simulink model "drone_estimator_angle_dynamics"  (R2024a)
settings: Solver=FixedStepAuto  StartTime=0.0  StopTime=30  FixedStep=0.001  RelTol=1e-3
InitFcn:
  | os = 0.15;
  | zeta = -log(os)/sqrt(pi^2+(log(os))^2);
  | ts = 0.2;
  | wn = 4/zeta/ts;
  | kx = wn^2 - 1;
  | kf = 2 * zeta * wn;
  | Kx = eye(2) * kx;
  | Kf = eye(2) * kf;
  | 
  | 
  | os_des = 0.1;
  | zeta_des = -log(os_des)/sqrt(pi^2+(log(os_des))^2);
  | ts_des = 1;
  | wn_des = 4/zeta_des/ts_des;
  | b_des = wn_des^2;
  | a_des = 2 * zeta_des * wn_des;
undefined symbols (not defined in the file or in its folder): e0_0, e1_0, e2_0, e3_0, q0, QP, vec
libraries: sharedtransform x12, dspsigops x12, sharedutil x6, simulink x3
(part 1 of 2)
settings Model: Creator=bemran  LastModifiedBy=bemran

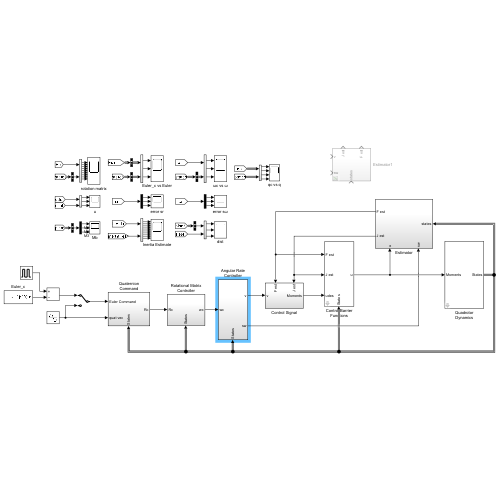
[thumbnail: Simulink's stored preview of the top-level diagram]
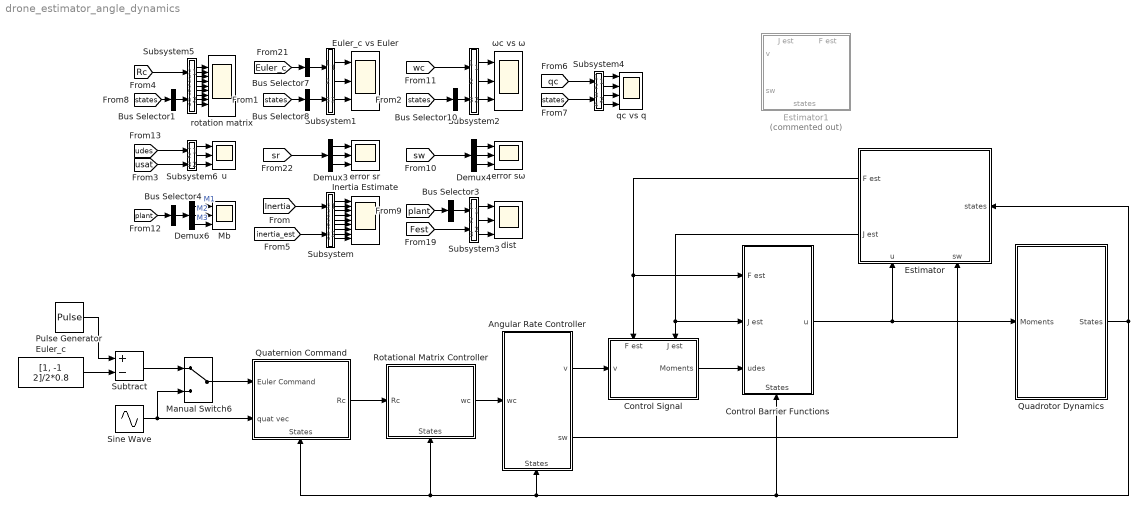
== system drone_estimator_angle_dynamics ==
  Angular Rate Controller : Subsystem
      settings: PortSchema="{\"entries\":[{\"content\":{\"sides\":[{\"content\":{\"connectorIds\":[\"In1\"]},\"type\":\"ConnectorPlacement.EquallySpacedRectSide\",\"uuid\":\"bc172b6d-1998-4b63-a77e-55c15233d681\"},{\"content\":{\"connectorIds\":[\"Out1\",\"Out2\"],\"side\":\"RIGHT\"},\"type\":\"ConnectorPlacement.EquallySpacedRectSide\",\"uuid\":\"e273a2d7-8de6-43d9-a3cd-224a066eb420\"},{\"content\":{\"side\":\"TOP\"},\"type\":\"ConnectorPlacement.EquallySpacedRectSide\",\"uuid\":\"072f3d67-5acb-4515-8061-1025c18e9c92\"},{\"content\":{\"connectorIds\":[\"In2\"],\"side\":\"BOTTOM\"},\"type\":\"ConnectorPlacement.EquallySpacedRectSide\",\"uuid\":\"23d2cd87-0863-4bc6-9ec0-2d909e89db59\"}]},\"type\":\"ConnectorPlacement.EquallySpacedConnector\",\"uuid\":\"0291006e-df7f-48c2-854b-3fa02a3c9ebe\"}],\"packageUris\":[\"http://schema.mathworks.com/mf0/Connector/R2020b\"],\"version\":\"1.0\"}"
  Bus Selector1 : BusSelector  OutputSignals=DCM_be  OutputAsBus=on
  Bus Selector10 : BusSelector  OutputSignals=w.p,w.q,w.r  OutputAsBus=on
  Bus Selector3 : BusSelector  OutputSignals=dist  OutputAsBus=on
  Bus Selector4 : BusSelector  OutputSignals=u  OutputAsBus=on
  Bus Selector7 : BusSelector  OutputSignals=ϕc,θc,Ψc  OutputAsBus=on
  Bus Selector8 : BusSelector  OutputSignals=Euler.ϕ,Euler.θ,Euler.Ψ  OutputAsBus=on
  Control Barrier Functions : Subsystem  mask{MaxU=30, MinU=-30, MaxW=20, MinW=-20}
      mask prompts: MaxU "Maximum Momentum"; MinU "Minimum Momentum"; MaxW "Maximum Omega"; MinW "Minimum Omega"
      settings: PortSchema="{\"entries\":[{\"content\":{\"sides\":[{\"content\":{\"connectorIds\":[\"In1\",\"In2\",\"In3\"]},\"type\":\"ConnectorPlacement.EquallySpacedRectSide\",\"uuid\":\"dcc8a69e-9139-493e-8673-5f35c41b34de\"},{\"content\":{\"connectorIds\":[\"Out1\"],\"side\":\"RIGHT\"},\"type\":\"ConnectorPlacement.EquallySpacedRectSide\",\"uuid\":\"2dca4313-3691-4a08-9138-e65173157107\"},{\"content\":{\"side\":\"TOP\"},\"type\":\"ConnectorPlacement.EquallySpacedRectSide\",\"uuid\":\"349ab802-a657-4b93-842b-98d2d831e594\"},{\"content\":{\"connectorIds\":[\"In4\"],\"side\":\"BOTTOM\"},\"type\":\"ConnectorPlacement.EquallySpacedRectSide\",\"uuid\":\"8ea90ba3-5825-4aab-a654-9f2643502d53\"}]},\"type\":\"ConnectorPlacement.EquallySpacedConnector\",\"uuid\":\"4208f7a9-c52c-44b5-9388-6b2af73cf8e5\"}],\"packageUris\":[\"http://schema.mathworks.com/mf0/Connector/R2020b\"],\"version\":\"1.0\"}"
      mask TypeOptions MaxU: MaxU/Value
      mask TypeOptions MinU: MinU/Value
      mask TypeOptions MaxW: MaxW/Value
      mask TypeOptions MinW: MinW/Value
  Control Signal : Subsystem
      settings: PortSchema="{\"entries\":[{\"content\":{\"sides\":[{\"content\":{\"connectorIds\":[\"In1\"]},\"type\":\"ConnectorPlacement.EquallySpacedRectSide\",\"uuid\":\"8e76b4e0-9a75-4e0d-89ba-89445e2fc413\"},{\"content\":{\"connectorIds\":[\"Out1\"],\"side\":\"RIGHT\"},\"type\":\"ConnectorPlacement.EquallySpacedRectSide\",\"uuid\":\"8c2e0e8a-5733-437d-85b2-5dcae92259bc\"},{\"content\":{\"connectorIds\":[\"In2\",\"In3\"],\"side\":\"TOP\"},\"type\":\"ConnectorPlacement.EquallySpacedRectSide\",\"uuid\":\"0f355bac-c390-4b16-a489-c47462c0e821\"},{\"content\":{\"side\":\"BOTTOM\"},\"type\":\"ConnectorPlacement.EquallySpacedRectSide\",\"uuid\":\"c09fe95f-7587-46e4-92c1-9bab0ec13c57\"}]},\"type\":\"ConnectorPlacement.EquallySpacedConnector\",\"uuid\":\"5b127af5-2db1-4950-aad7-ca3070de8172\"}],\"packageUris\":[\"http://schema.mathworks.com/mf0/Connector/R2020b\"],\"version\":\"1.0\"}"
  Demux3 : Demux  Outputs=3
  Demux4 : Demux  Outputs=3
  Demux6 : Demux  Outputs=3
  Estimator : Subsystem
      settings: PortSchema="{\"entries\":[{\"content\":{\"sides\":[{\"content\":{},\"type\":\"ConnectorPlacement.EquallySpacedRectSide\",\"uuid\":\"dd8d0a7b-0398-466a-94a7-19864dbb7504\"},{\"content\":{\"connectorIds\":[\"In2\",\"In3\"],\"side\":\"RIGHT\"},\"type\":\"ConnectorPlacement.EquallySpacedRectSide\",\"uuid\":\"1f79f4fb-283e-4db7-838d-a1872a06439d\"},{\"content\":{\"connectorIds\":[\"In1\"],\"side\":\"TOP\"},\"type\":\"ConnectorPlacement.EquallySpacedRectSide\",\"uuid\":\"5e0e8233-da53-4403-9876-3f6f01163ba4\"},{\"content\":{\"connectorIds\":[\"Out1\",\"Out2\"],\"side\":\"BOTTOM\"},\"type\":\"ConnectorPlacement.EquallySpacedRectSide\",\"uuid\":\"ef1fb064-42c9-4e33-ac14-a7a48f45da2d\"}]},\"type\":\"ConnectorPlacement.EquallySpacedConnector\",\"uuid\":\"c21bdc57-4e96-4c86-bff3-633ae446dfd3\"}],\"packageUris\":[\"http://schema.mathworks.com/mf0/Connector/R2020b\"],\"version\":\"1.0\"}"
  Estimator1 : Subsystem  Commented=on
      settings: PortSchema="{\"entries\":[{\"content\":{\"sides\":[{\"content\":{\"connectorIds\":[\"In1\",\"In2\"]},\"type\":\"ConnectorPlacement.EquallySpacedRectSide\",\"uuid\":\"dd8d0a7b-0398-466a-94a7-19864dbb7504\"},{\"content\":{\"side\":\"RIGHT\"},\"type\":\"ConnectorPlacement.EquallySpacedRectSide\",\"uuid\":\"1f79f4fb-283e-4db7-838d-a1872a06439d\"},{\"content\":{\"connectorIds\":[\"Out1\",\"Out2\"],\"side\":\"TOP\"},\"type\":\"ConnectorPlacement.EquallySpacedRectSide\",\"uuid\":\"5e0e8233-da53-4403-9876-3f6f01163ba4\"},{\"content\":{\"connectorIds\":[\"In3\"],\"side\":\"BOTTOM\"},\"type\":\"ConnectorPlacement.EquallySpacedRectSide\",\"uuid\":\"ef1fb064-42c9-4e33-ac14-a7a48f45da2d\"}]},\"type\":\"ConnectorPlacement.EquallySpacedConnector\",\"uuid\":\"c21bdc57-4e96-4c86-bff3-633ae446dfd3\"}],\"packageUris\":[\"http://schema.mathworks.com/mf0/Connector/R2020b\"],\"version\":\"1.0\"}"
  Euler_c : Constant  Value=[1, -1 2]/2*0.8
  Euler_c vs Euler : Scope  NumInputPorts=3
  Inertia Estimate : Scope  NumInputPorts=9
  Manual Switch6 : ManualSwitch
  Mb : Scope  NumInputPorts=3
  Pulse Generator : DiscretePulseGenerator  PulseType=Time based  Amplitude=[-1, -1, 4]*0.8  Period=[25, 37, 45]  PulseWidth=[60, 40, 50]  PhaseDelay=[0, 13, 8]
  Quadrotor Dynamics : Subsystem  mask{InertiaM=[1.7, 0.2, 0.3; 0.2, 2.4, 0.7; 0.3, 0.7, 3.2] + [QP.InertiaMatrix * 0 + diag([1.5,1.2,2]) + ones(3)*0.2]*0, EulerInitialValues=[1, 0.8, 1]*-pi/2, OmegaInitialValues=[-1;1; 1]*-1}
      mask prompts: InertiaM "Inertia Matrix"; EulerInitialValues "Euler Initial Values"; OmegaInitialValues "Omega Initial Values"
      mask TypeOptions InertiaM: Dynamics/Angular Velocity Dyanmics/InertiaMatrix
      mask TypeOptions EulerInitialValues: Dynamics/Quaternion Dynamics/EulerInitialValues
      mask TypeOptions OmegaInitialValues: Dynamics/Angular Velocity Dyanmics/OmegaInitialValues
      mask DialogControl Container4 Prompt: Parameters
      mask DialogControl Container5 Prompt: Initial Conditions
  Quaternion Command : Subsystem
      settings: PortSchema="{\"entries\":[{\"content\":{\"sides\":[{\"content\":{\"connectorIds\":[\"In1\",\"In2\"]},\"type\":\"ConnectorPlacement.EquallySpacedRectSide\",\"uuid\":\"ab38e5a5-80b4-4ab8-a53a-65892619af31\"},{\"content\":{\"connectorIds\":[\"Out1\"],\"side\":\"RIGHT\"},\"type\":\"ConnectorPlacement.EquallySpacedRectSide\",\"uuid\":\"8715b2e2-d98c-47a7-9943-c760a43dac77\"},{\"content\":{\"side\":\"TOP\"},\"type\":\"ConnectorPlacement.EquallySpacedRectSide\",\"uuid\":\"40574ceb-ae4a-44b3-ac35-a21b012f7856\"},{\"content\":{\"connectorIds\":[\"In3\"],\"side\":\"BOTTOM\"},\"type\":\"ConnectorPlacement.EquallySpacedRectSide\",\"uuid\":\"26ed6dc8-3652-4856-a0a2-f0a897d5f128\"}]},\"type\":\"ConnectorPlacement.EquallySpacedConnector\",\"uuid\":\"d4d113a2-0092-45e8-ae58-dde56ef36bed\"}],\"packageUris\":[\"http://schema.mathworks.com/mf0/Connector/R2020b\"],\"version\":\"1.0\"}"
  Rotational Matrix Controller : Subsystem
      settings: PortSchema="{\"entries\":[{\"content\":{\"sides\":[{\"content\":{\"connectorIds\":[\"In1\"]},\"type\":\"ConnectorPlacement.EquallySpacedRectSide\",\"uuid\":\"3d78e969-c8a0-4bae-8d29-4309eff7c33e\"},{\"content\":{\"connectorIds\":[\"Out1\"],\"side\":\"RIGHT\"},\"type\":\"ConnectorPlacement.EquallySpacedRectSide\",\"uuid\":\"5a76abcf-08d0-4f78-ba00-cefe271d19f3\"},{\"content\":{\"side\":\"TOP\"},\"type\":\"ConnectorPlacement.EquallySpacedRectSide\",\"uuid\":\"9a4251fd-9b0c-42f6-8a3e-81b1fbae2b4d\"},{\"content\":{\"connectorIds\":[\"In2\"],\"side\":\"BOTTOM\"},\"type\":\"ConnectorPlacement.EquallySpacedRectSide\",\"uuid\":\"0ec39cec-73e3-40ef-a15f-c71162c87a73\"}]},\"type\":\"ConnectorPlacement.EquallySpacedConnector\",\"uuid\":\"a6a66122-20c0-4355-ae71-2ed9e39c6f14\"}],\"packageUris\":[\"http://schema.mathworks.com/mf0/Connector/R2020b\"],\"version\":\"1.0\"}"
  Sine Wave : Sin  Amplitude=[1*pi;1*pi; 1*pi]/2  Frequency=[0.1, 0.05, 0.02]  Phase=[pi/6, pi/2, -pi/6]  SampleTime=0
  Subsystem : Subsystem
  Subsystem1 : Subsystem
  Subsystem2 : Subsystem
  Subsystem3 : Subsystem
  Subsystem4 : Subsystem
  Subsystem5 : Subsystem
  Subsystem6 : Subsystem
  Subtract : Sum  Inputs=+-
  dist : Scope  NumInputPorts=3
  error sr : Scope  NumInputPorts=3
  error sω : Scope  NumInputPorts=3
  qc vs q : Scope  NumInputPorts=4
  rotation matrix : Scope  NumInputPorts=9
  u : Scope  NumInputPorts=3
  ωc vs ω : Scope  NumInputPorts=3
  wires:
  Quaternion Command/1(Rc) -> Rotational Matrix Controller/1(Rc)
  Control Barrier Functions/1(u) -> Estimator/3(u), Quadrotor Dynamics/1(Moments)
  [sr] -> Demux3/1
  [states] -> Bus Selector10/1
  Subsystem2/1(Out1) -> ωc vs ω/1
  [wc] -> Subsystem2/1(wc)
  Demux6/3 -> Mb/3  "M3"
  Demux6/1 -> Mb/1  "M1"
  Demux6/2 -> Mb/2  "M2"
  Demux4/1 -> error sω/1
  Subsystem2/3(Out3) -> ωc vs ω/3
  [sw] -> Demux4/1
  Demux3/1 -> error sr/1
  Demux4/2 -> error sω/2
  Subsystem2/2(Out2) -> ωc vs ω/2
  Demux3/2 -> error sr/2
  Bus Selector4/1 -> Demux6/1
  Demux3/3 -> error sr/3
  Demux4/3 -> error sω/3
  [Fest] -> Subsystem3/2(fest)
  Subsystem3/1(Out1) -> dist/1
  Subsystem3/3(Out3) -> dist/3
  Subsystem3/2(Out2) -> dist/2
  [plant] -> Bus Selector3/1
  Control Signal/1(Moments) -> Control Barrier Functions/3(udes)
  Subsystem/1(Out1) -> Inertia Estimate/1
  Subsystem/2(Out2) -> Inertia Estimate/2
  Subsystem/3(Out3) -> Inertia Estimate/3
  Subsystem/4(Out4) -> Inertia Estimate/4
  Subsystem/5(Out5) -> Inertia Estimate/5
  Subsystem/6(Out6) -> Inertia Estimate/6
  Subsystem/7(Out7) -> Inertia Estimate/7
  Subsystem/8(Out8) -> Inertia Estimate/8
  Subsystem/9(Out9) -> Inertia Estimate/9
  [inertia_est] -> Subsystem/2(In6)
  [Euler_c] -> Bus Selector7/1
  [states] -> Bus Selector8/1
  Subsystem1/1(Out1) -> Euler_c vs Euler/1
  Subsystem1/2(Out2) -> Euler_c vs Euler/2
  Subsystem1/3(Out3) -> Euler_c vs Euler/3
  Bus Selector7/1 -> Subsystem1/1(Euler_c)
  Bus Selector8/1 -> Subsystem1/2(Euler)
  Bus Selector10/1 -> Subsystem2/2(w)
  Euler_c/1 -> Subtract/2
  Pulse Generator/1 -> Subtract/1
  Manual Switch6/1 -> Quaternion Command/1(Euler Command)
  Subtract/1 -> Manual Switch6/1
  Subsystem4/2(Out2) -> qc vs q/2
  Subsystem4/3(Out3) -> qc vs q/3
  [qc] -> Subsystem4/1(In1)
  Subsystem4/1(Out1) -> qc vs q/1
  [states] -> Subsystem4/2(In3)
  Subsystem4/4(Out4) -> qc vs q/4
  [states] -> Bus Selector1/1
  [Rc] -> Subsystem5/1(In4)
  Subsystem5/9(Out9) -> rotation matrix/9
  Subsystem5/8(Out8) -> rotation matrix/8
  Subsystem5/7(Out7) -> rotation matrix/7
  Subsystem5/6(Out6) -> rotation matrix/6
  Subsystem5/5(Out5) -> rotation matrix/5
  Subsystem5/4(Out4) -> rotation matrix/4
  Subsystem5/3(Out3) -> rotation matrix/3
  Subsystem5/2(Out2) -> rotation matrix/2
  Subsystem5/1(Out1) -> rotation matrix/1
  Bus Selector1/1 -> Subsystem5/2(In6)
  [Inertia] -> Subsystem/1(In4)
  Bus Selector3/1 -> Subsystem3/1(dist)
  [plant] -> Bus Selector4/1
  Sine Wave/1 -> Manual Switch6/2, Quaternion Command/2(quat vec)
  Estimator/2(J est) -> Control Signal/3(J est), Control Barrier Functions/2(J est)
  Estimator/1(F est) -> Control Signal/2(F est), Control Barrier Functions/1(F est)
  Rotational Matrix Controller/1(wc) -> Angular Rate Controller/1(wc)
  Quadrotor Dynamics/1(States) -> Estimator/1(states), Quaternion Command/3(States), Rotational Matrix Controller/2(States), Angular Rate Controller/2(States), Control Barrier Functions/4(States)
  Angular Rate Controller/1(v) -> Control Signal/1(v)
  Angular Rate Controller/2(sw) -> Estimator/2(sw)
  [usat] -> Subsystem6/2(u sat)
  Subsystem6/1(Out1) -> u/1
  Subsystem6/2(Out2) -> u/2
  Subsystem6/3(Out3) -> u/3
  [udes] -> Subsystem6/1(u)

== system drone_estimator_angle_dynamics/Angular Rate Controller ==
  wc : Inport
  In Bus Element : Inport  Port=2  PortName=States  Element=w
  Add : Sum
  Dynamic Surface Angular Rate Controller : Subsystem  mask{OmegaTimeConstant=20, PControllerGain=9, IControllerGain=4, DesiredAngularRateInitCond=zeros(3,1)}
      mask prompts: OmegaTimeConstant "Omega Time Constant"; PControllerGain "Propotional Controller Gain"; IControllerGain "Integral Controller Gain"; DesiredAngularRateInitCond "Desired Angular Rate Initial Condition"
      mask TypeOptions OmegaTimeConstant:
      | Angular Rate
      | Desired Dynamics/tau/Gain
      mask TypeOptions PControllerGain: P gain/Gain
      mask TypeOptions IControllerGain: I gain/Gain
      mask TypeOptions DesiredAngularRateInitCond:
      | Angular Rate
      | Desired Dynamics/Desired Angular
      | Rate Integaration/InitialCondition
  Manual Switch : ManualSwitch  CurrentSetting=0
  Pulse Generator : DiscretePulseGenerator  PulseType=Time based  Amplitude=[3, -3, 3]*0.8  Period=[20, 20, 20]  PulseWidth=50  PhaseDelay=[0 7 13]
  Sine Wave : Sin  Amplitude=[1*pi;1*pi; 1*pi]  Frequency=[0.1, 0.05, 0.02]*10  Phase=[pi/6, pi/2, -pi/6]  SampleTime=0
  v : Outport
  sw : Outport  Port=2
  wires:
  Sine Wave/1 -> Add/2
  Manual Switch/1 -> Dynamic Surface Angular Rate Controller/1(wc)
  Dynamic Surface Angular Rate Controller/2(sw) -> sw/1
  Pulse Generator/1 -> Add/1
  Dynamic Surface Angular Rate Controller/1(v) -> v/1
  Add/1 -> Manual Switch/1
  wc/1 -> Manual Switch/2
  In Bus Element/1 -> Dynamic Surface Angular Rate Controller/2(w)

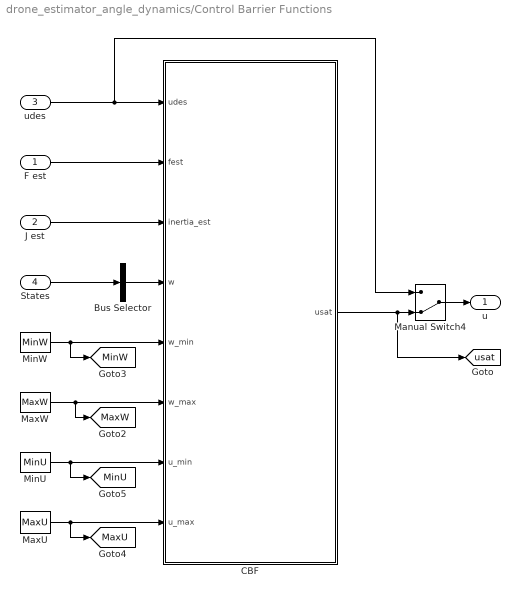
== system drone_estimator_angle_dynamics/Control Barrier Functions ==
  F est : Inport
  J est : Inport  Port=2
  udes : Inport  Port=3
  States : Inport  Port=4
  Bus Selector : BusSelector  OutputSignals=w.p,w.q,w.r  OutputAsBus=on
  CBF : MATLAB Function  TreatAsAtomicUnit=on
  Manual Switch4 : ManualSwitch  CurrentSetting=0
  MaxU : Constant  Value=MaxU
  MaxW : Constant  Value=MaxW
  MinU : Constant  Value=MinU
  MinW : Constant  Value=MinW
  u : Outport
  tag scope: MaxU=global, MaxW=global, MinU=global, MinW=global, usat=global
  wires:
  J est/1 -> CBF/3(inertia_est)
  MaxW/1 -> [MaxW], CBF/6(w_max)
  MinW/1 -> [MinW], CBF/5(w_min)
  F est/1 -> CBF/2(fest)
  MinU/1 -> [MinU], CBF/7(u_min)
  MaxU/1 -> [MaxU], CBF/8(u_max)
  Bus Selector/1 -> CBF/4(w)
  States/1 -> Bus Selector/1
  CBF/1(usat) -> [usat], Manual Switch4/2
  udes/1 -> Manual Switch4/1, CBF/1(udes)
  Manual Switch4/1 -> u/1

== system drone_estimator_angle_dynamics/Control Signal ==
  v : Inport
  F est : Inport  Port=2
  J est : Inport  Port=3
  Product : Product  Inputs=**  Multiplication=Matrix(*)
  Sum1 : Sum  Inputs=|+-
  Moments : Outport
  tag scope: udes=global
  wires:
  Sum1/1 -> [udes], Moments/1
  F est/1 -> Sum1/2
  Product/1 -> Sum1/1
  v/1 -> Product/2
  J est/1 -> Product/1

== system drone_estimator_angle_dynamics/Estimator ==
  states : Inport
  sw : Inport  Port=2
  u : Inport  Port=3
  Add : Sum
  Constant : Constant  Value=zeros(3,1)
  Gain : Gain  Gain=0.3
  Inertia Estimation : Subsystem  mask{gamma=QP.InertiaMatrixGamma*5, MaxEstiamtedTheta=QP.InertiaMatrixMax*0 + 3*eye(3) + ones(3), MinEstiamtedTheta=QP.InertiaMatrixMin*0 + eye(3)*0.01, eps=0.01, InertiaInitialCondition=eye(3) + ones(3)*0.1}
      mask prompts: MaxEstiamtedTheta "Maximum Estiamted Theta"; MinEstiamtedTheta "Minimum Estiamted Theta"; eps "Epsilon Estiamted Theta"; InertiaInitialCondition "Inertia Initial Condition"
      mask TypeOptions gamma: gama/Gain
      mask TypeOptions MaxEstiamtedTheta: θ Max/Value
      mask TypeOptions MinEstiamtedTheta: θ Min/Value
      mask TypeOptions eps: eps/Value
      mask TypeOptions InertiaInitialCondition: θ estimate/InitialCondition
      mask DialogControl Container Prompt: Estimation Paraemter
  Manual Switch : ManualSwitch
  Manual Switch1 : ManualSwitch  CurrentSetting=0
  Model Predictor : Subsystem
      settings: PortSchema="{\"entries\":[{\"content\":{\"sides\":[{\"content\":{\"connectorIds\":[\"Out1\",\"Out2\"]},\"type\":\"ConnectorPlacement.EquallySpacedRectSide\",\"uuid\":\"6e6569c2-bc7f-4167-ae98-e66125c9e1e3\"},{\"content\":{\"connectorIds\":[\"In1\",\"In2\",\"In3\"],\"side\":\"RIGHT\"},\"type\":\"ConnectorPlacement.EquallySpacedRectSide\",\"uuid\":\"af0deaad-808c-4137-9b9d-c847525b3dac\"},{\"content\":{\"side\":\"TOP\"},\"type\":\"ConnectorPlacement.EquallySpacedRectSide\",\"uuid\":\"ed017cdd-fa89-4299-a174-caff2025e69e\"}]},\"type\":\"ConnectorPlacement.EquallySpacedConnector\",\"uuid\":\"feb2a9a1-0b16-4155-b32e-177a30695464\"}],\"packageUris\":[\"http://schema.mathworks.com/mf0/Connector/R2020b\"],\"version\":\"1.0\"}"
  Model Predictor1 : Subsystem  Commented=on
      settings: PortSchema="{\"entries\":[{\"content\":{\"sides\":[{\"content\":{\"connectorIds\":[\"Out1\",\"Out2\"]},\"type\":\"ConnectorPlacement.EquallySpacedRectSide\",\"uuid\":\"6e6569c2-bc7f-4167-ae98-e66125c9e1e3\"},{\"content\":{\"connectorIds\":[\"In1\",\"In2\",\"In3\",\"In4\"],\"side\":\"RIGHT\"},\"type\":\"ConnectorPlacement.EquallySpacedRectSide\",\"uuid\":\"af0deaad-808c-4137-9b9d-c847525b3dac\"},{\"content\":{\"side\":\"TOP\"},\"type\":\"ConnectorPlacement.EquallySpacedRectSide\",\"uuid\":\"ed017cdd-fa89-4299-a174-caff2025e69e\"}]},\"type\":\"ConnectorPlacement.EquallySpacedConnector\",\"uuid\":\"feb2a9a1-0b16-4155-b32e-177a30695464\"}],\"packageUris\":[\"http://schema.mathworks.com/mf0/Connector/R2020b\"],\"version\":\"1.0\"}"
  F est : Outport
  J est : Outport  Port=2
  tag scope: inertia_est=global
  wires:
  Model Predictor/1(er) -> Add/1
  Inertia Estimation/1("  θ est") -> Manual Switch/1
  [Inertia] -> Manual Switch/2
  Model Predictor/2(F est) -> F est/1
  Manual Switch/1 -> Model Predictor/3(J est), [inertia_est], J est/1
  states/1 -> Model Predictor/1(x)
  u/1 -> Model Predictor/2(u), Inertia Estimation/1(u)
  sw/1 -> Gain/1
  Gain/1 -> Manual Switch1/2
  Constant/1 -> Manual Switch1/1
  Manual Switch1/1 -> Add/2
  Add/1 -> Inertia Estimation/2(e)

== system drone_estimator_angle_dynamics/Estimator1 ==
  v : Inport
  sw : Inport  Port=2
  states : Inport  Port=3
  Add : Sum
  Constant : Constant  Value=zeros(3,1)
  Gain : Gain  Gain=0.3
  Inertia Estimation : Subsystem  mask{gamma=QP.InertiaMatrixGamma*1, MaxEstiamtedTheta=QP.InertiaMatrixMax*0 + 3*eye(3) + ones(3)*0.5, MinEstiamtedTheta=QP.InertiaMatrixMin*0 + eye(3)*0.01, eps=0.01, InertiaInitialCondition=ones(3)*0.3 + eye(3)}
      mask prompts: MaxEstiamtedTheta "Maximum Estiamted Theta"; MinEstiamtedTheta "Minimum Estiamted Theta"; eps "Epsilon Estiamted Theta"; InertiaInitialCondition "Inertia Initial Condition"
      mask TypeOptions gamma: gama/Gain
      mask TypeOptions MaxEstiamtedTheta: θ Max/Value
      mask TypeOptions MinEstiamtedTheta: θ Min/Value
      mask TypeOptions eps: eps/Value
      mask TypeOptions InertiaInitialCondition: θ estimate/InitialCondition
      mask DialogControl Container Prompt: Estimation Paraemter
  Manual Switch : ManualSwitch
  Manual Switch1 : ManualSwitch  CurrentSetting=0
  Model Predictor : Subsystem
      settings: PortSchema="{\"entries\":[{\"content\":{\"sides\":[{\"content\":{\"connectorIds\":[\"Out1\",\"Out2\"]},\"type\":\"ConnectorPlacement.EquallySpacedRectSide\",\"uuid\":\"6e6569c2-bc7f-4167-ae98-e66125c9e1e3\"},{\"content\":{\"connectorIds\":[\"In1\",\"In2\"],\"side\":\"RIGHT\"},\"type\":\"ConnectorPlacement.EquallySpacedRectSide\",\"uuid\":\"af0deaad-808c-4137-9b9d-c847525b3dac\"},{\"content\":{\"side\":\"TOP\"},\"type\":\"ConnectorPlacement.EquallySpacedRectSide\",\"uuid\":\"ed017cdd-fa89-4299-a174-caff2025e69e\"}]},\"type\":\"ConnectorPlacement.EquallySpacedConnector\",\"uuid\":\"feb2a9a1-0b16-4155-b32e-177a30695464\"}],\"packageUris\":[\"http://schema.mathworks.com/mf0/Connector/R2020b\"],\"version\":\"1.0\"}"
  Model Predictor1 : Subsystem  Commented=on
      settings: PortSchema="{\"entries\":[{\"content\":{\"sides\":[{\"content\":{\"connectorIds\":[\"Out1\",\"Out2\"]},\"type\":\"ConnectorPlacement.EquallySpacedRectSide\",\"uuid\":\"6e6569c2-bc7f-4167-ae98-e66125c9e1e3\"},{\"content\":{\"connectorIds\":[\"In1\",\"In2\",\"In3\",\"In4\"],\"side\":\"RIGHT\"},\"type\":\"ConnectorPlacement.EquallySpacedRectSide\",\"uuid\":\"af0deaad-808c-4137-9b9d-c847525b3dac\"},{\"content\":{\"side\":\"TOP\"},\"type\":\"ConnectorPlacement.EquallySpacedRectSide\",\"uuid\":\"ed017cdd-fa89-4299-a174-caff2025e69e\"}]},\"type\":\"ConnectorPlacement.EquallySpacedConnector\",\"uuid\":\"feb2a9a1-0b16-4155-b32e-177a30695464\"}],\"packageUris\":[\"http://schema.mathworks.com/mf0/Connector/R2020b\"],\"version\":\"1.0\"}"
  J est : Outport
  F est : Outport  Port=2
  tag scope: inertia_est=global
  wires:
  Add/1 -> Inertia Estimation/2(e)
  Manual Switch1/1 -> Add/2
  Constant/1 -> Manual Switch1/1
  Gain/1 -> Manual Switch1/2
  sw/1 -> Gain/1
  v/1 -> Inertia Estimation/1(v), Model Predictor/2(v)
  states/1 -> Model Predictor/1(x)
  Manual Switch/1 -> J est/1, [inertia_est]
  Model Predictor/2(F est) -> F est/1
  [Inertia] -> Manual Switch/2
  Inertia Estimation/1("  θ est") -> Manual Switch/1
  Model Predictor/1(er) -> Add/1

== system drone_estimator_angle_dynamics/Quadrotor Dynamics ==
  Moments : Inport  OutDataTypeStr=double
  Disturbance Generator : Subsystem
  Dynamics : Subsystem
  To Workspace : ToWorkspace  VariableName=states  SaveFormat=Timeseries  SampleTime=-1
  To Workspace1 : ToWorkspace  VariableName=plant  SaveFormat=Timeseries  SampleTime=-1
  States : Outport
  tag scope: plant=global, states=global
  wires:
  Moments/1 -> Dynamics/1(Moments)
  Dynamics/1(Plant) -> [plant], To Workspace1/1
  Dynamics/2(States) -> [states], Disturbance Generator/1(states), States/1, To Workspace/1
  Disturbance Generator/1(dist) -> Dynamics/2(Dist)

== system drone_estimator_angle_dynamics/Quaternion Command ==
  Euler Command : Inport
  quat vec : Inport  Port=2
  States : Inport  Port=3
  Filtering Command Signal : Subsystem  mask{RollRange=0.5, RollRisingSlewLimit=pi, RollFallingSlewLimit=-pi, YawRange=0.5, YawRisingSlewLimit=pi, YawFallingSlewLimit=-pi, PitchRange=0.5, PitchRisingSlewLimit=pi, PitchFallingSlewLimit=-pi}
      mask prompts: RollRange "Roll Saturation Range"; RollRisingSlewLimit "Roll Rising Slew Rate"; RollFallingSlewLimit "Roll Falling Slew Rate"; YawRange "Yaw Saturation Range"; YawRisingSlewLimit "Yaw Rising Slew Rate"; YawFallingSlewLimit "Yaw Falling Slew Rate"; PitchRange "Pitch Saturation Range"; PitchRisingSlewLimit "Pitch Rising Slew Rate"; PitchFallingSlewLimit "Pitch Falling Slew Rate"
      mask TypeOptions RollRange: Roll Dynamic Sat/Range
      mask TypeOptions RollRisingSlewLimit: Roll Rate Limiter/RisingSlewLimit
      mask TypeOptions RollFallingSlewLimit: Roll Rate Limiter/FallingSlewLimit
      mask TypeOptions YawRange: Yaw Dynamic Sat/Range
      mask TypeOptions YawRisingSlewLimit: Yaw Rate Limiter/RisingSlewLimit
      mask TypeOptions YawFallingSlewLimit: Yaw Rate Limiter/FallingSlewLimit
      mask TypeOptions PitchRange: Pitch Dynamic Sat/Range
      mask TypeOptions PitchRisingSlewLimit: Pitch Rate Limiter/RisingSlewLimit
      mask TypeOptions PitchFallingSlewLimit: Pitch Rate Limiter/FallingSlewLimit
      mask DialogControl Container4 Prompt: Roll
      mask DialogControl Container3 Prompt: Pitch
      mask DialogControl Container5 Prompt: Yaw
  Manual Switch : ManualSwitch
  Manual Switch2 : ManualSwitch
  Rotation Interpolation : Subsystem
  Scope1 : Scope
  Sine Wave1 : Sin  Amplitude=pi  Frequency=[0.1]  Phase=[-pi/2]  SampleTime=0
  "States " : InportShadow  Port=3
  ToGo : Subsystem
  quaternion : Subsystem
  to Rotation Mat : Subsystem
  Rc : Outport
  tag scope: Rc=global
  wires:
  Sine Wave1/1 -> quaternion/1(angle)
  quat vec/1 -> quaternion/2(vec)
  to Rotation Mat/1(rot) -> Manual Switch2/1
  quaternion/1(rot) -> Manual Switch2/2
  Manual Switch2/1 -> Manual Switch/1, Rotation Interpolation/1(DCM)
  Rotation Interpolation/1(Rot) -> Manual Switch/2
  States/1 -> Rotation Interpolation/2(States)
  Manual Switch/1 -> Scope1/1, Rc/1, [Rc]
  "States "/1 -> Filtering Command Signal/2(States)
  Euler Command/1 -> ToGo/1(DCM), Filtering Command Signal/1(Command)
  Filtering Command Signal/1(Filtered) -> to Rotation Mat/1(Euler)

== system drone_estimator_angle_dynamics/Rotational Matrix Controller ==
  Rc : Inport
  In Bus Element : Inport  Port=2  PortName=States  Element=DCM_be
  Quaternion Dynamics : Subsystem  mask{InitialCondition=eye(3,3), DesiredRotaionDynamciGain=20}
      mask prompts: InitialCondition "Simulink:blkprm_prompts:IntegratorInitCond"; DesiredRotaionDynamciGain "Desired Rotaion Dynamci Gain"
      mask TypeOptions InitialCondition:
      | Rotaion
      | Integration/InitialCondition
      mask TypeOptions DesiredRotaionDynamciGain:
      | Desired Rotaion
      | Dynamic Gain /Gain
      mask DialogControl InitialCondition Prompt: Initial condition:
  Rotational Controller : Subsystem  mask{RotationControlGain=diag([1,1,1]) * 5}
      mask prompts: RotationControlGain "Rotation Control Gain"
      mask TypeOptions RotationControlGain: Kr/Value
      mask DialogControl ParameterGroupVar Prompt: Control Gain
  wc : Outport
  wires:
  Rotational Controller/1(wc) -> wc/1
  Quaternion Dynamics/1(Rd) -> Rotational Controller/1(Rd)
  Rc/1 -> Quaternion Dynamics/1(R)
  Quaternion Dynamics/2(Rd_dot) -> Rotational Controller/2(Rd_dot)
  In Bus Element/1 -> Rotational Controller/3(Rot)

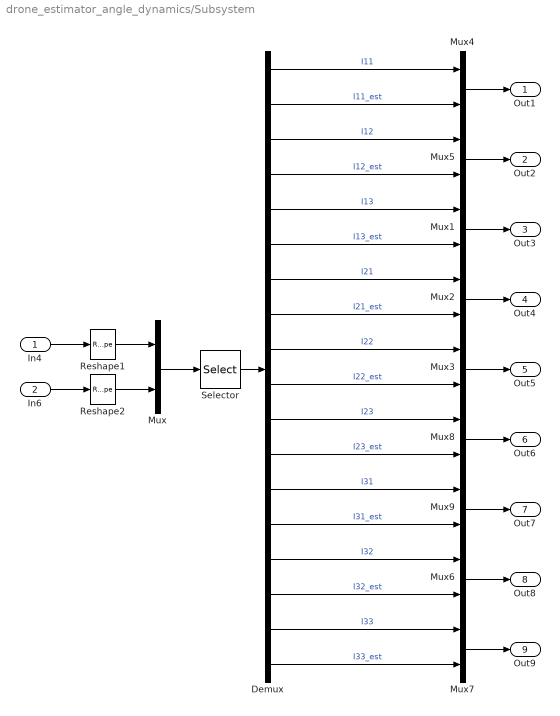
== system drone_estimator_angle_dynamics/Subsystem ==
  In4 : Inport
  In6 : Inport  Port=2
  Demux : Demux  Outputs=18
  Mux{,1..9} (10 alike) : Mux  Inputs=2
  Reshape1 : Reshape  OutputDimensionality=Column vector (2-D)
  Reshape2 : Reshape  OutputDimensionality=Column vector (2-D)
  Selector : Selector  InputPortWidth=18  IndexOptions=Index vector (dialog)  Indices=[1 10 2 11 3 12 4 13 5 14 6 15 7 16 8 17 9 18]  OutputSizes=1
  Out1 : Outport
  Out2 : Outport  Port=2
  Out3 : Outport  Port=3
  Out4 : Outport  Port=4
  Out5 : Outport  Port=5
  Out6 : Outport  Port=6
  Out7 : Outport  Port=7
  Out8 : Outport  Port=8
  Out9 : Outport  Port=9
  wires:
  Mux8/1 -> Out6/1
  Mux/1 -> Selector/1
  Mux2/1 -> Out4/1
  Reshape2/1 -> Mux/2
  Mux9/1 -> Out7/1
  Mux1/1 -> Out3/1
  In4/1 -> Reshape1/1
  Demux/2 -> Mux4/2  "I11_est"
  In6/1 -> Reshape2/1
  Demux/1 -> Mux4/1  "I11"
  Reshape1/1 -> Mux/1
  Demux/3 -> Mux5/1  "I12"
  Selector/1 -> Demux/1
  Mux3/1 -> Out5/1
  Demux/4 -> Mux5/2  "I12_est"
  Demux/5 -> Mux1/1  "I13"
  Demux/6 -> Mux1/2  "I13_est"
  Demux/7 -> Mux2/1  "I21"
  Mux4/1 -> Out1/1
  Demux/8 -> Mux2/2  "I21_est"
  Demux/9 -> Mux3/1  "I22"
  Demux/10 -> Mux3/2  "I22_est"
  Demux/11 -> Mux8/1  "I23"
  Mux5/1 -> Out2/1
  Demux/12 -> Mux8/2  "I23_est"
  Demux/13 -> Mux9/1  "I31"
  Demux/14 -> Mux9/2  "I31_est"
  Demux/15 -> Mux6/1  "I32"
  Mux6/1 -> Out8/1
  Demux/16 -> Mux6/2  "I32_est"
  Demux/17 -> Mux7/1  "I33"
  Demux/18 -> Mux7/2  "I33_est"
  Mux7/1 -> Out9/1

== system drone_estimator_angle_dynamics/Subsystem1 ==
  Euler_c : Inport
  Euler : Inport  Port=2
  Demux2 : Demux  Outputs=6
  Mux{,9..11} (4 alike) : Mux  Inputs=2
  Selector : Selector  InputPortWidth=6  IndexOptions=Index vector (dialog)  Indices=[1 4 2 5 3 6]  OutputSizes=1
  Out1 : Outport
  Out2 : Outport  Port=2
  Out3 : Outport  Port=3
  wires:
  Mux9/1 -> Out1/1
  Mux11/1 -> Out3/1
  Mux10/1 -> Out2/1
  Euler/1 -> Mux/2
  Euler_c/1 -> Mux/1
  Demux2/1 -> Mux9/1  "ϕc"
  Demux2/2 -> Mux9/2  "ϕ"
  Demux2/3 -> Mux10/1  "θc"
  Demux2/4 -> Mux10/2  "θ"
  Demux2/5 -> Mux11/1  "Ψc"
  Demux2/6 -> Mux11/2  "Ψ"
  Selector/1 -> Demux2/1
  Mux/1 -> Selector/1

== system drone_estimator_angle_dynamics/Subsystem2 ==
  wc : Inport
  w : Inport  Port=2
  Demux2 : Demux  Outputs=6
  Mux{,9..11} (4 alike) : Mux  Inputs=2
  Selector : Selector  InputPortWidth=6  IndexOptions=Index vector (dialog)  Indices=[1 4 2 5 3 6]  OutputSizes=1
  Out1 : Outport
  Out2 : Outport  Port=2
  Out3 : Outport  Port=3
  wires:
  Demux2/6 -> Mux11/2  "r"
  Demux2/5 -> Mux11/1  "rc"
  Demux2/4 -> Mux10/2  "q"
  Demux2/3 -> Mux10/1  "qc"
  Demux2/2 -> Mux9/2  "p"
  Demux2/1 -> Mux9/1  "pc"
  Mux10/1 -> Out2/1
  Mux11/1 -> Out3/1
  Mux9/1 -> Out1/1
  wc/1 -> Mux/1
  Selector/1 -> Demux2/1
  w/1 -> Mux/2
  Mux/1 -> Selector/1

== system drone_estimator_angle_dynamics/Subsystem3 ==
  dist : Inport
  fest : Inport  Port=2
  Demux2 : Demux  Outputs=6
  Mux{,9..11} (4 alike) : Mux  Inputs=2
  Selector : Selector  InputPortWidth=6  IndexOptions=Index vector (dialog)  Indices=[1 4 2 5 3 6]  OutputSizes=1
  Out1 : Outport
  Out2 : Outport  Port=2
  Out3 : Outport  Port=3
  wires:
  Demux2/6 -> Mux11/2  "f3"
  Demux2/5 -> Mux11/1  "d3"
  Demux2/4 -> Mux10/2  "f2"
  Demux2/3 -> Mux10/1  "d2"
  Demux2/2 -> Mux9/2  "f1"
  Demux2/1 -> Mux9/1  "d1"
  dist/1 -> Mux/1
  fest/1 -> Mux/2
  Mux10/1 -> Out2/1
  Mux11/1 -> Out3/1
  Mux9/1 -> Out1/1
  Mux/1 -> Selector/1
  Selector/1 -> Demux2/1

== system drone_estimator_angle_dynamics/Subsystem4 ==
  In1 : Inport
  In3 : Inport  Port=2
  Bus Selector2 : BusSelector  OutputSignals=Quat.q0,Quat.vec
  Demux : Demux  Outputs=3
  Demux2 : Demux  Outputs=8
  Mux{1..2,9..11} (5 alike) : Mux  Inputs=2
  Mux3 : Mux
  Selector : Selector  InputPortWidth=8  IndexOptions=Index vector (dialog)  Indices=[1 5 2 6 3 7 4 8]  OutputSizes=1
  Out1 : Outport
  Out2 : Outport  Port=2
  Out3 : Outport  Port=3
  Out4 : Outport  Port=4
  wires:
  Mux9/1 -> Out1/1
  Mux10/1 -> Out2/1
  Mux11/1 -> Out3/1
  Mux1/1 -> Out4/1
  In1/1 -> Mux2/1  "qc"
  Demux2/1 -> Mux9/1  "qc0"
  Demux2/2 -> Mux9/2  "q0"
  Demux2/4 -> Mux10/2  "q1"
  Demux2/3 -> Mux10/1  "qc1"
  Demux2/6 -> Mux11/2  "q2"
  Demux2/5 -> Mux11/1  "qc2"
  Demux2/8 -> Mux1/2  "q3"
  Demux2/7 -> Mux1/1  "qc3"
  Selector/1 -> Demux2/1
  Bus Selector2/1 -> Mux3/1  "<q0>"
  In3/1 -> Bus Selector2/1  "q"
  Bus Selector2/2 -> Demux/1  "<vec>"
  Demux/2 -> Mux3/3
  Demux/1 -> Mux3/2
  Demux/3 -> Mux3/4
  Mux3/1 -> Mux2/2
  Mux2/1 -> Selector/1

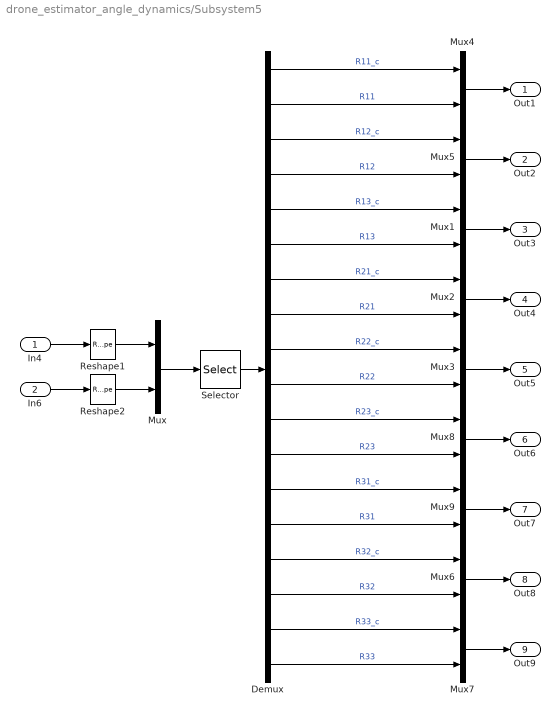
== system drone_estimator_angle_dynamics/Subsystem5 ==
  In4 : Inport
  In6 : Inport  Port=2
  Demux : Demux  Outputs=18
  Mux{,1..9} (10 alike) : Mux  Inputs=2
  Reshape1 : Reshape  OutputDimensionality=Column vector (2-D)
  Reshape2 : Reshape  OutputDimensionality=Column vector (2-D)
  Selector : Selector  InputPortWidth=18  IndexOptions=Index vector (dialog)  Indices=[1 10 2 11 3 12 4 13 5 14 6 15 7 16 8 17 9 18]  OutputSizes=1
  Out1 : Outport
  Out2 : Outport  Port=2
  Out3 : Outport  Port=3
  Out4 : Outport  Port=4
  Out5 : Outport  Port=5
  Out6 : Outport  Port=6
  Out7 : Outport  Port=7
  Out8 : Outport  Port=8
  Out9 : Outport  Port=9
  wires:
  Mux7/1 -> Out9/1
  Demux/18 -> Mux7/2  "R33"
  Demux/17 -> Mux7/1  "R33_c"
  Demux/16 -> Mux6/2  "R32"
  Mux6/1 -> Out8/1
  Demux/15 -> Mux6/1  "R32_c"
  Demux/14 -> Mux9/2  "R31"
  Demux/13 -> Mux9/1  "R31_c"
  Demux/12 -> Mux8/2  "R23"
  Mux5/1 -> Out2/1
  Demux/11 -> Mux8/1  "R23_c"
  Demux/10 -> Mux3/2  "R22"
  Demux/9 -> Mux3/1  "R22_c"
  Demux/8 -> Mux2/2  "R21"
  Mux4/1 -> Out1/1
  Demux/7 -> Mux2/1  "R21_c"
  Demux/6 -> Mux1/2  "R13"
  Demux/5 -> Mux1/1  "R13_c"
  Demux/4 -> Mux5/2  "R12"
  Mux3/1 -> Out5/1
  Selector/1 -> Demux/1
  Demux/3 -> Mux5/1  "R12_c"
  Reshape1/1 -> Mux/1
  Demux/1 -> Mux4/1  "R11_c"
  In6/1 -> Reshape2/1
  Demux/2 -> Mux4/2  "R11"
  In4/1 -> Reshape1/1
  Mux1/1 -> Out3/1
  Mux9/1 -> Out7/1
  Reshape2/1 -> Mux/2
  Mux2/1 -> Out4/1
  Mux/1 -> Selector/1
  Mux8/1 -> Out6/1

== system drone_estimator_angle_dynamics/Subsystem6 ==
  u : Inport
  u sat : Inport  Port=2
  Demux2 : Demux  Outputs=6
  Mux{,9..11} (4 alike) : Mux  Inputs=2
  Selector : Selector  InputPortWidth=6  IndexOptions=Index vector (dialog)  Indices=[1 4 2 5 3 6]  OutputSizes=1
  Out1 : Outport
  Out2 : Outport  Port=2
  Out3 : Outport  Port=3
  wires:
  Mux/1 -> Selector/1
  Selector/1 -> Demux2/1
  Demux2/6 -> Mux11/2  "u3 sat"
  Demux2/5 -> Mux11/1  "u3"
  Demux2/4 -> Mux10/2  "u2 sat"
  Demux2/3 -> Mux10/1  "u2"
  Demux2/2 -> Mux9/2  "u1 sat"
  Demux2/1 -> Mux9/1  "u1"
  u/1 -> Mux/1
  u sat/1 -> Mux/2
  Mux10/1 -> Out2/1
  Mux11/1 -> Out3/1
  Mux9/1 -> Out1/1

== system drone_estimator_angle_dynamics/Angular Rate Controller/Dynamic Surface Angular Rate Controller ==
  wc : Inport
  w : Inport  Port=2
  Angular Rate Desired Dynamics : Subsystem
  I gain : Gain  Gain=IControllerGain
  Integrator : Integrator
  P gain : Gain  Gain=PControllerGain
  Subtract : Sum  Inputs=|+-
  Sum : Sum  Inputs=--+
  v : Outport
  sw : Outport  Port=2
  tag scope: sw=global, wc=global
  wires:
  Angular Rate Desired Dynamics/2(wd dot) -> Sum/3  "wd dot"
  P gain/1 -> Sum/1  "Sw * Kpw"
  Angular Rate Desired Dynamics/1(wd) -> Subtract/2  "wd"
  w/1 -> Subtract/1
  Subtract/1 -> P gain/1, [sw], sw/1, Integrator/1
  wc/1 -> [wc], Angular Rate Desired Dynamics/1(wc)
  Sum/1 -> v/1
  Integrator/1 -> I gain/1
  I gain/1 -> Sum/2  "(Sw)_i * Kiw"

== system drone_estimator_angle_dynamics/Estimator/Inertia Estimation ==
  u : Inport
  e : Inport  Port=2
  MATLAB Function : MATLAB Function  TreatAsAtomicUnit=on
  Reshape : Reshape  OutputDimensionality=Column vector (2-D)
  Reshape1 : Reshape  OutputDimensionality=Column vector (2-D)
  Scope : Scope
  eps : Constant  Value=eps
  gama : Gain  Gain=gamma
  θ Max : Constant  Value=MaxEstiamtedTheta
  θ Min : Constant  Value=MinEstiamtedTheta
  θ estimate : Integrator  InitialCondition=InertiaInitialCondition  LimitOutput=on  UpperSaturationLimit=MaxEstiamtedTheta  LowerSaturationLimit=MinEstiamtedTheta
  "  θ est" : Outport
  wires:
  gama/1 -> θ estimate/1
  θ Max/1 -> MATLAB Function/4(est_max)
  θ Min/1 -> MATLAB Function/5(est_min)
  θ estimate/1 -> Scope/1, MATLAB Function/1(est), "  θ est"/1
  MATLAB Function/1(est_dot) -> gama/1
  u/1 -> Reshape/1
  e/1 -> Reshape1/1
  Reshape/1 -> MATLAB Function/3(v)
  Reshape1/1 -> MATLAB Function/2(e)
  eps/1 -> MATLAB Function/6(eps)

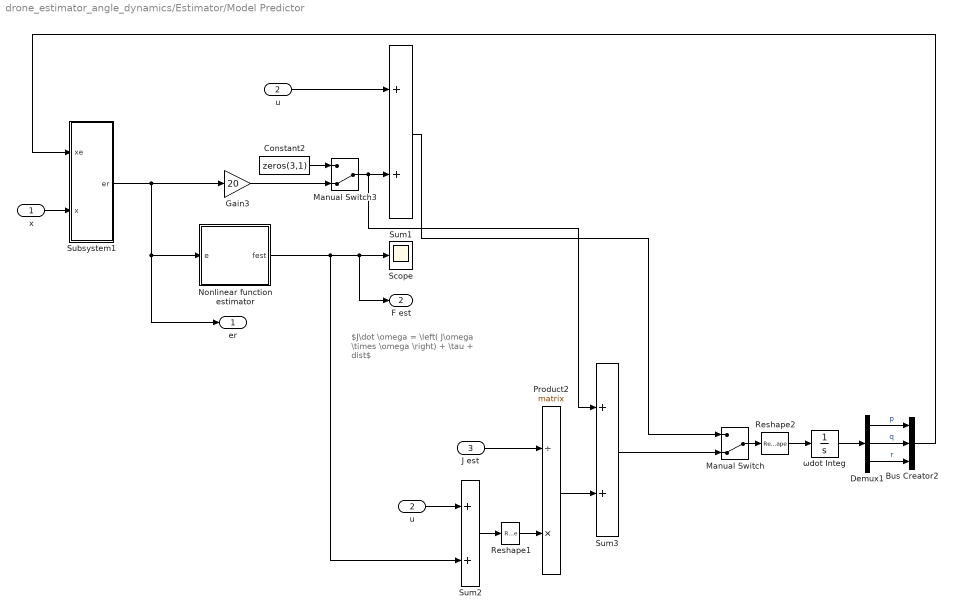
== system drone_estimator_angle_dynamics/Estimator/Model Predictor ==
  note: $J\dot \omega = \left( J\omega \times \omega \right) + \tau + dist$
  x : Inport
  u : Inport  Port=2
  J est : Inport  Port=3
  Bus Creator2 : BusCreator  Inputs=3
  Constant2 : Constant  Value=zeros(3,1)
  Demux1 : Demux  Outputs=3
  Gain3 : Gain  Gain=20
  Manual Switch : ManualSwitch  CurrentSetting=0
  Manual Switch3 : ManualSwitch  CurrentSetting=0
  Nonlinear function estimator : Subsystem
  Product2 : Product  Inputs=/*  Multiplication=Matrix(*)  SaturateOnIntegerOverflow=on  OutDataTypeStr=Inherit: Same as first input
  Reshape1 : Reshape  OutputDimensionality=Column vector (2-D)
  Reshape2 : Reshape
  Scope : Scope
  Subsystem1 : Subsystem
  Sum1 : Sum  SaturateOnIntegerOverflow=on
  Sum2 : Sum  SaturateOnIntegerOverflow=on
  Sum3 : Sum  SaturateOnIntegerOverflow=on
  "u " : InportShadow  Port=2
  ωdot Integ : Integrator  ContinuousStateAttributes={'p', 'q', 'r'}
  er : Outport
  F est : Outport  Port=2
  wires:
  Reshape2/1 -> ωdot Integ/1
  ωdot Integ/1 -> Demux1/1
  Demux1/3 -> Bus Creator2/3  "r"
  Demux1/2 -> Bus Creator2/2  "q"
  Demux1/1 -> Bus Creator2/1  "p"
  Sum1/1 -> Manual Switch/1
  x/1 -> Subsystem1/2(x)
  Subsystem1/1(er) -> Gain3/1, er/1, Nonlinear function estimator/1(e)
  Manual Switch3/1 -> Sum3/1, Sum1/2
  Gain3/1 -> Manual Switch3/2
  Constant2/1 -> Manual Switch3/1
  u/1 -> Sum1/1
  Nonlinear function estimator/1(fest) -> Sum2/2, F est/1, Scope/1
  Bus Creator2/1 -> Subsystem1/1(xe)
  Sum2/1 -> Reshape1/1
  J est/1 -> Product2/1
  Reshape1/1 -> Product2/2
  Sum3/1 -> Manual Switch/2
  Manual Switch/1 -> Reshape2/1
  "u "/1 -> Sum2/1
  Product2/1 -> Sum3/2

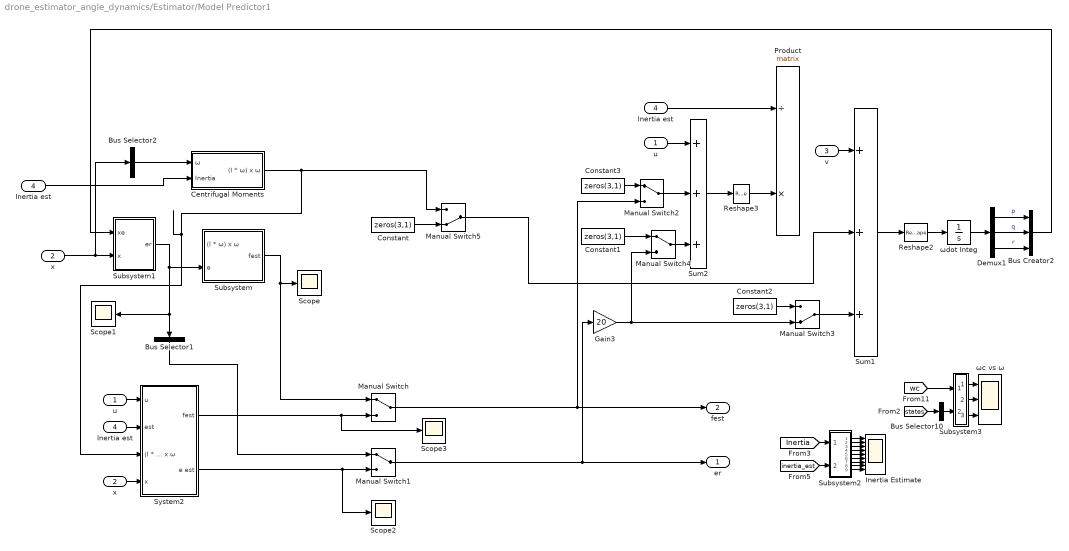
== system drone_estimator_angle_dynamics/Estimator/Model Predictor1 ==
  u : Inport
  x : Inport  Port=2
  v : Inport  Port=3
  Inertia est : Inport  Port=4
  Bus Creator2 : BusCreator  Inputs=3
  Bus Selector1 : BusSelector  OutputSignals=ep,eq,er  OutputAsBus=on
  Bus Selector10 : BusSelector  OutputSignals=w.p,w.q,w.r  OutputAsBus=on
  Bus Selector2 : BusSelector  OutputSignals=w.p,w.q,w.r  OutputAsBus=on
  Centrifugal Moments : Subsystem
  Constant{,1..3} (4 alike) : Constant  Value=zeros(3,1)
  Demux1 : Demux  Outputs=3
  Gain3 : Gain  Gain=20
  Inertia Estimate : Scope  NumInputPorts=9
  "Inertia est " : InportShadow  Port=4
  "Inertia est  " : InportShadow  Port=4
  Manual Switch{,1..2,4} (4 alike) : ManualSwitch
  Manual Switch3 : ManualSwitch  CurrentSetting=0
  Manual Switch5 : ManualSwitch  CurrentSetting=0
  Product : Product  Inputs=/*  Multiplication=Matrix(*)  SaturateOnIntegerOverflow=on  OutDataTypeStr=Inherit: Same as first input
  Reshape2 : Reshape
  Reshape3 : Reshape  OutputDimensionality=Column vector (2-D)
  Scope{,1..3} (4 alike) : Scope
  Subsystem : Subsystem
  Subsystem1 : Subsystem
  Subsystem2 : Subsystem
  Subsystem3 : Subsystem
  Sum1 : Sum  Inputs=+++  SaturateOnIntegerOverflow=on
  Sum2 : Sum  Inputs=+++  SaturateOnIntegerOverflow=on
  System2 : Subsystem
  "u " : InportShadow
  "x " : InportShadow  Port=2
  ωc vs ω : Scope  NumInputPorts=3
  ωdot Integ : Integrator  ContinuousStateAttributes={'p', 'q', 'r'}
  er : Outport
  fest : Outport  Port=2
  wires:
  Bus Creator2/1 -> Subsystem1/1(xe)
  Centrifugal Moments/1((I * ω) x ω) -> Manual Switch5/1, System2/3((I * ω) x ω)
  Bus Selector2/1 -> Centrifugal Moments/1(ω)
  Inertia est/1 -> Centrifugal Moments/2(Inertia)
  Manual Switch/1 -> Manual Switch2/2, fest/1
  Manual Switch2/1 -> Sum2/2
  v/1 -> Sum1/1
  Manual Switch5/1 -> Sum1/2
  Constant3/1 -> Manual Switch2/1
  Constant/1 -> Manual Switch5/2
  Subsystem3/2(Out2) -> ωc vs ω/2
  Subsystem3/3(Out3) -> ωc vs ω/3
  [wc] -> Subsystem3/1(In1)
  Subsystem3/1(Out1) -> ωc vs ω/1
  [states] -> Bus Selector10/1
  Bus Selector10/1 -> Subsystem3/2(In2)
  Constant2/1 -> Manual Switch3/1
  Constant1/1 -> Manual Switch4/1
  Manual Switch4/1 -> Sum2/3
  Gain3/1 -> Manual Switch3/2, Manual Switch4/2
  Manual Switch3/1 -> Sum1/3
  Manual Switch1/1 -> Gain3/1, er/1
  Subsystem2/5(Out5) -> Inertia Estimate/5
  Subsystem2/9(Out9) -> Inertia Estimate/9
  Subsystem2/2(Out2) -> Inertia Estimate/2
  Subsystem2/3(Out3) -> Inertia Estimate/3
  Subsystem2/1(Out1) -> Inertia Estimate/1
  [Inertia] -> Subsystem2/1(In4)
  Subsystem2/8(Out8) -> Inertia Estimate/8
  Subsystem2/4(Out4) -> Inertia Estimate/4
  Subsystem2/7(Out7) -> Inertia Estimate/7
  Subsystem2/6(Out6) -> Inertia Estimate/6
  [inertia_est] -> Subsystem2/2(In6)
  Bus Selector1/1 -> Manual Switch1/1
  System2/2(e est) -> Manual Switch1/2, Scope2/1
  System2/1(fest) -> Manual Switch/2, Scope3/1
  "x "/1 -> System2/4(x)
  "u "/1 -> System2/1(u)
  "Inertia est  "/1 -> System2/2(est)
  Subsystem1/1(er) -> Subsystem/2(e), Bus Selector1/1, Scope1/1
  x/1 -> Subsystem1/2(x), Bus Selector2/1
  Subsystem/1(fest) -> Scope/1, Manual Switch/1
  "Inertia est "/1 -> Product/1
  Sum1/1 -> Reshape2/1
  u/1 -> Sum2/1
  Reshape3/1 -> Product/2
  Demux1/1 -> Bus Creator2/1  "p"
  Sum2/1 -> Reshape3/1
  Demux1/2 -> Bus Creator2/2  "q"
  Demux1/3 -> Bus Creator2/3  "r"
  ωdot Integ/1 -> Demux1/1
  Reshape2/1 -> ωdot Integ/1

== system drone_estimator_angle_dynamics/Estimator1/Inertia Estimation ==
  v : Inport
  e : Inport  Port=2
  MATLAB Function : MATLAB Function  TreatAsAtomicUnit=on
  Reshape : Reshape  OutputDimensionality=Column vector (2-D)
  Reshape1 : Reshape  OutputDimensionality=Column vector (2-D)
  Scope : Scope
  eps : Constant  Value=eps
  gama : Gain  Gain=gamma
  θ Max : Constant  Value=MaxEstiamtedTheta
  θ Min : Constant  Value=MinEstiamtedTheta
  θ estimate : Integrator  InitialCondition=InertiaInitialCondition  LimitOutput=on  UpperSaturationLimit=MaxEstiamtedTheta  LowerSaturationLimit=MinEstiamtedTheta
  "  θ est" : Outport
  wires:
  eps/1 -> MATLAB Function/6(eps)
  Reshape1/1 -> MATLAB Function/2(e)
  Reshape/1 -> MATLAB Function/3(v)
  e/1 -> Reshape1/1
  v/1 -> Reshape/1
  MATLAB Function/1(est_dot) -> gama/1
  θ estimate/1 -> "  θ est"/1, MATLAB Function/1(est), Scope/1
  θ Min/1 -> MATLAB Function/5(est_min)
  θ Max/1 -> MATLAB Function/4(est_max)
  gama/1 -> θ estimate/1

== system drone_estimator_angle_dynamics/Estimator1/Model Predictor ==
  x : Inport
  v : Inport  Port=2
  Bus Creator2 : BusCreator  Inputs=3
  Constant2 : Constant  Value=zeros(3,1)
  Demux1 : Demux  Outputs=3
  Gain3 : Gain  Gain=20
  Manual Switch3 : ManualSwitch  CurrentSetting=0
  Nonlinear function estimator : Subsystem
  Reshape2 : Reshape
  Scope : Scope
  Subsystem1 : Subsystem
  Sum1 : Sum  SaturateOnIntegerOverflow=on
  ωdot Integ : Integrator  ContinuousStateAttributes={'p', 'q', 'r'}
  er : Outport
  F est : Outport  Port=2
  wires:
  Bus Creator2/1 -> Subsystem1/1(xe)
  Nonlinear function estimator/1(fest) -> Scope/1, F est/1
  v/1 -> Sum1/1
  Constant2/1 -> Manual Switch3/1
  Gain3/1 -> Manual Switch3/2
  Manual Switch3/1 -> Sum1/2
  Subsystem1/1(er) -> Nonlinear function estimator/1(e), er/1, Gain3/1
  x/1 -> Subsystem1/2(x)
  Sum1/1 -> Reshape2/1
  Demux1/1 -> Bus Creator2/1  "p"
  Demux1/2 -> Bus Creator2/2  "q"
  Demux1/3 -> Bus Creator2/3  "r"
  ωdot Integ/1 -> Demux1/1
  Reshape2/1 -> ωdot Integ/1

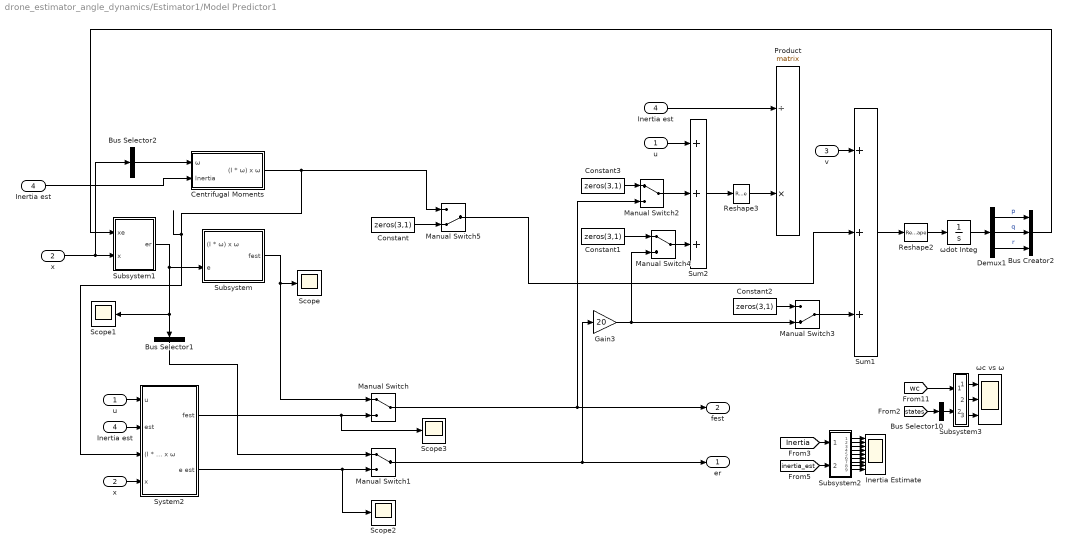
== system drone_estimator_angle_dynamics/Estimator1/Model Predictor1 ==
  u : Inport
  x : Inport  Port=2
  v : Inport  Port=3
  Inertia est : Inport  Port=4
  Bus Creator2 : BusCreator  Inputs=3
  Bus Selector1 : BusSelector  OutputSignals=ep,eq,er  OutputAsBus=on
  Bus Selector10 : BusSelector  OutputSignals=w.p,w.q,w.r  OutputAsBus=on
  Bus Selector2 : BusSelector  OutputSignals=w.p,w.q,w.r  OutputAsBus=on
  Centrifugal Moments : Subsystem
  Constant{,1..3} (4 alike) : Constant  Value=zeros(3,1)
  Demux1 : Demux  Outputs=3
  Gain3 : Gain  Gain=20
  Inertia Estimate : Scope  NumInputPorts=9
  "Inertia est " : InportShadow  Port=4
  "Inertia est  " : InportShadow  Port=4
  Manual Switch{,1..2,4} (4 alike) : ManualSwitch
  Manual Switch3 : ManualSwitch  CurrentSetting=0
  Manual Switch5 : ManualSwitch  CurrentSetting=0
  Product : Product  Inputs=/*  Multiplication=Matrix(*)  SaturateOnIntegerOverflow=on  OutDataTypeStr=Inherit: Same as first input
  Reshape2 : Reshape
  Reshape3 : Reshape  OutputDimensionality=Column vector (2-D)
  Scope{,1..3} (4 alike) : Scope
  Subsystem : Subsystem
  Subsystem1 : Subsystem
  Subsystem2 : Subsystem
  Subsystem3 : Subsystem
  Sum1 : Sum  Inputs=+++  SaturateOnIntegerOverflow=on
  Sum2 : Sum  Inputs=+++  SaturateOnIntegerOverflow=on
  System2 : Subsystem
  "u " : InportShadow
  "x " : InportShadow  Port=2
  ωc vs ω : Scope  NumInputPorts=3
  ωdot Integ : Integrator  ContinuousStateAttributes={'p', 'q', 'r'}
  er : Outport
  fest : Outport  Port=2
  wires:
  Reshape2/1 -> ωdot Integ/1
  ωdot Integ/1 -> Demux1/1
  Demux1/3 -> Bus Creator2/3  "r"
  Demux1/2 -> Bus Creator2/2  "q"
  Sum2/1 -> Reshape3/1
  Demux1/1 -> Bus Creator2/1  "p"
  Reshape3/1 -> Product/2
  u/1 -> Sum2/1
  Sum1/1 -> Reshape2/1
  "Inertia est "/1 -> Product/1
  Subsystem/1(fest) -> Manual Switch/1, Scope/1
  x/1 -> Bus Selector2/1, Subsystem1/2(x)
  Subsystem1/1(er) -> Scope1/1, Bus Selector1/1, Subsystem/2(e)
  "Inertia est  "/1 -> System2/2(est)
  "u "/1 -> System2/1(u)
  "x "/1 -> System2/4(x)
  System2/1(fest) -> Scope3/1, Manual Switch/2
  System2/2(e est) -> Scope2/1, Manual Switch1/2
  Bus Selector1/1 -> Manual Switch1/1
  [inertia_est] -> Subsystem2/2(In6)
  Subsystem2/6(Out6) -> Inertia Estimate/6
  Subsystem2/7(Out7) -> Inertia Estimate/7
  Subsystem2/4(Out4) -> Inertia Estimate/4
  Subsystem2/8(Out8) -> Inertia Estimate/8
  [Inertia] -> Subsystem2/1(In4)
  Subsystem2/1(Out1) -> Inertia Estimate/1
  Subsystem2/3(Out3) -> Inertia Estimate/3
  Subsystem2/2(Out2) -> Inertia Estimate/2
  Subsystem2/9(Out9) -> Inertia Estimate/9
  Subsystem2/5(Out5) -> Inertia Estimate/5
  Manual Switch1/1 -> er/1, Gain3/1
  Manual Switch3/1 -> Sum1/3
  Gain3/1 -> Manual Switch4/2, Manual Switch3/2
  Manual Switch4/1 -> Sum2/3
  Constant1/1 -> Manual Switch4/1
  Constant2/1 -> Manual Switch3/1
  Bus Selector10/1 -> Subsystem3/2(In2)
  [states] -> Bus Selector10/1
  Subsystem3/1(Out1) -> ωc vs ω/1
  [wc] -> Subsystem3/1(In1)
  Subsystem3/3(Out3) -> ωc vs ω/3
  Subsystem3/2(Out2) -> ωc vs ω/2
  Constant/1 -> Manual Switch5/2
  Constant3/1 -> Manual Switch2/1
  Manual Switch5/1 -> Sum1/2
  v/1 -> Sum1/1
  Manual Switch2/1 -> Sum2/2
  Manual Switch/1 -> fest/1, Manual Switch2/2
  Inertia est/1 -> Centrifugal Moments/2(Inertia)
  Bus Selector2/1 -> Centrifugal Moments/1(ω)
  Centrifugal Moments/1((I * ω) x ω) -> System2/3((I * ω) x ω), Manual Switch5/1
  Bus Creator2/1 -> Subsystem1/1(xe)

== system drone_estimator_angle_dynamics/Quadrotor Dynamics/Disturbance Generator ==
  states : Inport
  Bus Selector : BusSelector  OutputSignals=w.p,w.q,w.r  OutputAsBus=on
  Gain1 : Gain  Gain=0.5
  Manual Switch : ManualSwitch  CurrentSetting=0
  Pulse Generator : DiscretePulseGenerator  PulseType=Time based  Amplitude=[1, -1, 2]*2  Period=[50, 67, 87]  PulseWidth=[30, 80, 50]
  Sin : Trigonometry
  Square2 : Math  Operator=square
  zero dist : Constant  Value=[0;0;0]
  dist : Outport
  wires:
  Gain1/1 -> Sin/1
  states/1 -> Bus Selector/1
  Bus Selector/1 -> Gain1/1
  zero dist/1 -> Manual Switch/2
  Pulse Generator/1 -> Manual Switch/1
  Manual Switch/1 -> dist/1

== system drone_estimator_angle_dynamics/Quadrotor Dynamics/Dynamics ==
  Moments : Inport  OutDataTypeStr=double
  Dist : Inport  Port=2  OutDataTypeStr=double
  Angular Velocity Dyanmics : Subsystem  mask{OmegaInitialValues=OmegaInitialValues, InertiaMatrix=InertiaM}
      mask prompts: OmegaInitialValues "Omega Initial Values"; InertiaMatrix "Inertia Matrix"
      mask TypeOptions OmegaInitialValues: ωdot Integ/InitialCondition
      mask TypeOptions InertiaMatrix: Inertia Matrix/Value
  Constant1 : Constant  Value=zeros(3,1)
  Manual Switch1 : ManualSwitch
  Mixer : Subsystem  Commented=on  mask{ThustForceCoefficient=QP.Gu}
      mask prompts: ThustForceCoefficient "Thust and Force Coefficient"
      mask TypeOptions ThustForceCoefficient: Constant/Value
  Quaternion Dynamics : Subsystem  mask{EulerInitialValues=EulerInitialValues}
      mask prompts: EulerInitialValues "Euler Initial Values"
  Bus Element Out1 : Outport  PortName=Plant  Element=fc
  Bus Element Out2 : Outport  PortName=Plant  Element=dist
  Bus Element Out9 : Outport  PortName=Plant  Element=u
  Bus Element Out4 : Outport  Port=2  PortName=States  Element=DCM_be
  Bus Element Out5 : Outport  Port=2  PortName=States  Element=Quat
  Bus Element Out6 : Outport  Port=2  PortName=States  Element=Euler
  Bus Element Out7 : Outport  Port=2  PortName=States  Element=w
  Bus Element Out8 : Outport  Port=2  PortName=States  Element=wdot
  wires:
  Angular Velocity Dyanmics/1(ω) -> Bus Element Out7/1, Quaternion Dynamics/1(ω)
  Moments/1 -> Bus Element Out9/1, Angular Velocity Dyanmics/1(Moments)
  Manual Switch1/1 -> Bus Element Out2/1, Angular Velocity Dyanmics/2(Dist)
  Angular Velocity Dyanmics/3(fc) -> Bus Element Out1/1
  Angular Velocity Dyanmics/2(ωdot) -> Bus Element Out8/1
  Dist/1 -> Manual Switch1/2
  Constant1/1 -> Manual Switch1/1
  Quaternion Dynamics/3(Euler) -> Bus Element Out6/1
  Quaternion Dynamics/2(Quat) -> Bus Element Out5/1
  Quaternion Dynamics/1(DCM_be) -> Bus Element Out4/1
